simulink model "sampleModel160"  (R2021b)
settings: Solver=VariableStepAuto  StartTime=0.0  StopTime=10.0  RelTol=1e-3
undefined symbols (not defined in the file or in its folder): DiscIntNeverNeededParam, Newton, Raphson
libraries: simulink x16, slpidlib x1
settings Model: Creator=user  LastModifiedBy=user

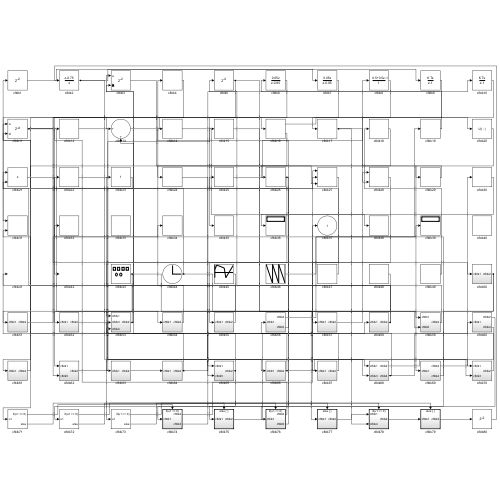
[thumbnail: Simulink's stored preview of the top-level diagram]
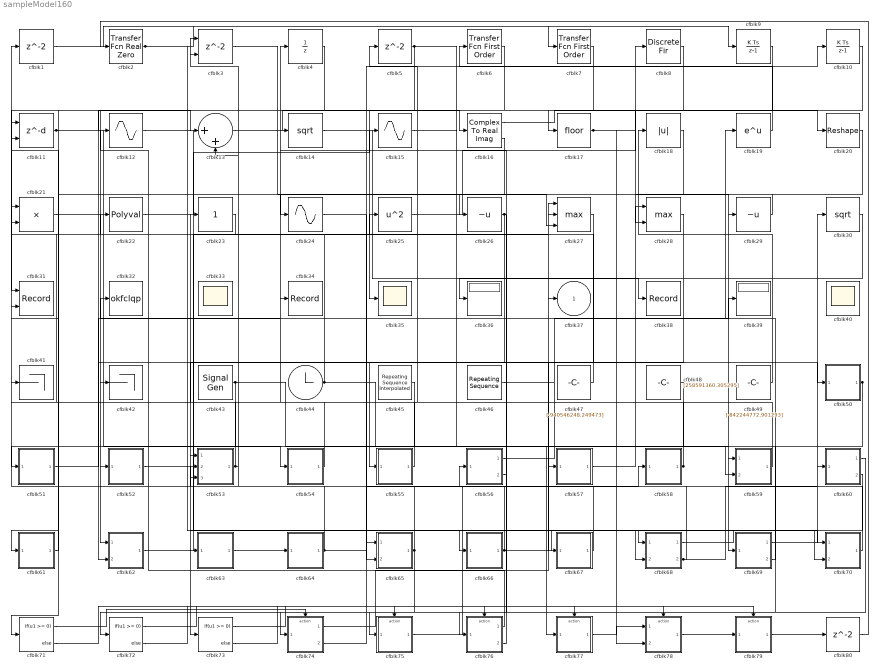
== system sampleModel160 ==
  cfblk1 : Delay  SampleTime=1
  cfblk10 : DiscreteIntegrator  ICPrevOutput=DiscIntNeverNeededParam  ICPrevScaledInput=DiscIntNeverNeededParam
  cfblk11 : Delay  DelayLengthSource=Input port  SampleTime=1
      settings: InputPortMap=u0,p1
  cfblk12 : Sin  TimeSource=Use external signal  SampleTime=0
  cfblk13 : Sum  Inputs=|++
  cfblk14 : Sqrt  SaturateOnIntegerOverflow=on
  cfblk15 : Sin  TimeSource=Use external signal  SampleTime=0
  cfblk16 : ComplexToRealImag
  cfblk17 : Rounding
  cfblk18 : Abs
  cfblk19 : Math  SaturateOnIntegerOverflow=on
  cfblk2 : simulink/Discrete/Transfer Fcn Real Zero  ZeroZ=0.75  ICPrevInput=0.0  DoSatur=off
      settings: SourceProductBaseCode=SL
  cfblk20 : Reshape
  cfblk21 : Product  Inputs=**
  cfblk22 : Polyval  Coefs=[ +2.081618890e-019, -1.441693666e-014, +4.719686976e-010, -8.536869453e-006, +1.621573104e-001, -8.087801117e+001 ]
  cfblk23 : simulink/Math Operations/Slider Gain  gain=1  low=0  high=2
  cfblk24 : Sin  TimeSource=Use external signal  SampleTime=0
  cfblk25 : Math  Operator=square  SaturateOnIntegerOverflow=on
  cfblk26 : UnaryMinus
  cfblk27 : MinMax  Function=max  Inputs=3
  cfblk28 : MinMax  Function=max  Inputs=2
  cfblk29 : UnaryMinus
  cfblk3 : Delay  ShowEnablePort=on  SampleTime=1
      settings: InputPortMap=u0,e6
  cfblk30 : Sqrt  SaturateOnIntegerOverflow=on
  cfblk31 : Record  FileSettingsInternal="{\"entries\":[{\"content\":{\"excelSettings\":{\"content\":{},\"type\":\"Streamout.ExcelSettings\"}},\"type\":\"Streamout.FileSettingStorage\",\"uuid\":\"c413c589-d2ce-436c-aaba-4ffc6c089058\"}],\"packageUris\":[\"http://schema.mathworks.com/mf0/streamout_blocks/R2020a\"],\"version\":\"1.0\"}"  Layout=[1 1]  SignalsInternal="{\"entries\":[{\"content\":{\"signals\":[{\"content\":{\"blockPath\":[\"sampleModel160/cfblk31\"],\"channel\":[],\"dimensions\":[1],\"domain\":\"sampleModel160/cfblk31\",\"lineColor\":\"#a2142f\",\"plots\":[1],\"port\":1,\"sid\":[\"\"],\"signalID\":6037,\"signalName\":\"cfblk10\"},\"type\":\"RecordBlkView.Signal\",\"uuid\":\"72857fe4-462d-486d-a3e4-3c395ee845b6\"},{\"content\":{\"blockPath\":[\"sampleModel160/cfblk31\"],\"channel\":[],\"dimensions\":[1],\"domain\":\"sampleModel160/cfblk31\",\"lineColor\":\"#139fff\",\"plots\":[1],\"port\":2,\"sid\":[\"\"],\"signalID\":6041,\"signalName\":\"cfblk61\"},\"type\":\"RecordBlkView.Signal\",\"uuid\":\"d5c775f5-053a-4779-9e26-d54423a1e3c8\"}]},\"type\":\"RecordBlkView.InputSignals\",\"uuid\":\"1cc1dd8b-340d-4e21-9a8e-fa59a4d45196\"}],\"packageUris\":[\"http://schema.mathworks.com/mf0/streamout_blocks/R2020a\"],\"version\":\"1.0\"}"  VisualizationBindings="{\"xyplotplugin\":{\"info\":[{\"series\":[{\"bindingParametersList\":[{\"parameter\":\"X-Axis\",\"signalID\":6037,\"signalName\":\"cfblk10\"},{\"parameter\":\"Y-Axis\",\"signalID\":6041,\"signalName\":\"cfblk61\"}],\"seriesID\":10105}],\"subplotID\":1}]}}"  CompatibilityTag=XY
  cfblk32 : ToWorkspace  VariableName=okfclqp  SaveFormat=Timeseries  SampleTime=-1
  cfblk33 : Scope
      settings: Floating=on
  cfblk34 : Record  FileSettingsInternal="{\"entries\":[{\"content\":{\"excelSettings\":{\"content\":{},\"type\":\"Streamout.ExcelSettings\"}},\"type\":\"Streamout.FileSettingStorage\",\"uuid\":\"c9e76eac-59f3-42f9-ba3c-d666261c6b06\"}],\"packageUris\":[\"http://schema.mathworks.com/mf0/streamout_blocks/R2020a\"],\"version\":\"1.0\"}"  SignalsInternal="{\"entries\":[{\"content\":{\"signals\":[{\"content\":{\"blockPath\":[\"sampleModel160/cfblk34\"],\"channel\":[],\"dimensions\":[1],\"domain\":\"sampleModel160/cfblk34\",\"lineColor\":\"#fe330a\",\"plots\":[1],\"port\":1,\"sid\":[\"\"],\"signalID\":6045,\"signalName\":\"cfblk51\"},\"type\":\"RecordBlkView.Signal\",\"uuid\":\"385a5dff-ef78-469a-be59-ea6837f228a9\"}]},\"type\":\"RecordBlkView.InputSignals\",\"uuid\":\"b764ceec-8da9-4fc6-845a-cebcb7dbad93\"}],\"packageUris\":[\"http://schema.mathworks.com/mf0/streamout_blocks/R2020a\"],\"version\":\"1.0\"}"  VisualizationBindings="{\"sparklinesplugin\":{\"info\":[{\"bindingParametersList\":[],\"subplotID\":1}]}}"
  cfblk35 : Scope
  cfblk36 : Display
  cfblk38 : Record  FileSettingsInternal="{\"entries\":[{\"content\":{\"excelSettings\":{\"content\":{},\"type\":\"Streamout.ExcelSettings\"}},\"type\":\"Streamout.FileSettingStorage\",\"uuid\":\"a9748414-4318-452a-bfbb-77e6d7b29a13\"}],\"packageUris\":[\"http://schema.mathworks.com/mf0/streamout_blocks/R2020a\"],\"version\":\"1.0\"}"  SignalsInternal="{\"entries\":[{\"content\":{\"signals\":[{\"content\":{\"blockPath\":[\"sampleModel160/cfblk38\"],\"channel\":[],\"dimensions\":[1],\"domain\":\"sampleModel160/cfblk38\",\"lineColor\":\"#22b573\",\"plots\":[1],\"port\":1,\"sid\":[\"\"],\"signalID\":6049,\"signalName\":\"cfblk14\"},\"type\":\"RecordBlkView.Signal\",\"uuid\":\"85378120-5b17-4b37-8955-e146c021a7fe\"}]},\"type\":\"RecordBlkView.InputSignals\",\"uuid\":\"a0d2f558-881a-48b2-8250-b54130961238\"}],\"packageUris\":[\"http://schema.mathworks.com/mf0/streamout_blocks/R2020a\"],\"version\":\"1.0\"}"  VisualizationBindings="{\"sparklinesplugin\":{\"info\":[{\"bindingParametersList\":[],\"subplotID\":1}]}}"
  cfblk39 : Display
  cfblk4 : UnitDelay  HasFrameUpgradeWarning=on
  cfblk40 : Scope
      settings: Floating=on
  cfblk41 : Terminator
  cfblk42 : Terminator
  cfblk43 : SignalGenerator  Amplitude=[899162175.269200]
  cfblk44 : Clock
  cfblk45 : simulink/Sources/Repeating Sequence Interpolated  OutValues=[358173877.356189, 804234155.488900, 502386956.729002, -523743488.961026, 763410355.711706]  TimeValues=[0 0.1 0.5 0.6 1].'  LookUpMeth=Interpolation-Use End Values  tsamp=0.01  OutMin=[]  OutMax=[]  OutDataTypeStr=double  OutputDataTypeScalingMode=double  OutDataType=fixdt(0,8)  OutScaling=2^-10
  cfblk46 : simulink/Sources/Repeating Sequence  rep_seq_t=[0 2]  rep_seq_y=[661275798.341106, -980251664.687721]
  cfblk47 : Constant  Value=[-940546248.249473]  SampleTime=1
  cfblk48 : Constant  Value=[258591360.305295]  SampleTime=1
  cfblk49 : Constant  Value=[-842244772.901293]  SampleTime=1
  cfblk5 : Delay  SampleTime=1
  cfblk50 : Subsystem
  cfblk51 : Subsystem
  cfblk52 : Subsystem
  cfblk53 : Subsystem
  cfblk54 : Subsystem
  cfblk55 : Subsystem
  cfblk56 : Subsystem
  cfblk57 : Subsystem
  cfblk58 : Subsystem
  cfblk59 : Subsystem
  cfblk6 : simulink/Discrete/Transfer Fcn First Order  PoleZ=0.95  ICPrevOutput=0.0  DoSatur=off
  cfblk60 : Subsystem
  cfblk61 : Subsystem
  cfblk62 : Subsystem
  cfblk63 : Subsystem
  cfblk64 : Subsystem
  cfblk65 : Subsystem
  cfblk66 : Subsystem
  cfblk67 : Subsystem
  cfblk68 : Subsystem
  cfblk69 : Subsystem
  cfblk7 : simulink/Discrete/Transfer Fcn First Order  PoleZ=0.95  ICPrevOutput=0.0  DoSatur=off
  cfblk70 : Subsystem
  cfblk71 : If  IfExpression=u1 >= 0  SampleTime=1
  cfblk72 : If  IfExpression=u1 >= 0  SampleTime=1
  cfblk73 : If  IfExpression=u1 >= 0  SampleTime=1
  cfblk74 : Subsystem  TreatAsAtomicUnit=on
  cfblk75 : Subsystem  TreatAsAtomicUnit=on
  cfblk76 : Subsystem  TreatAsAtomicUnit=on
  cfblk77 : Subsystem  TreatAsAtomicUnit=on
  cfblk78 : Subsystem  TreatAsAtomicUnit=on
  cfblk79 : Subsystem  TreatAsAtomicUnit=on
  cfblk8 : DiscreteFir  SampleTime=1
  cfblk80 : Delay  SampleTime=1
  cfblk9 : DiscreteIntegrator  ICPrevOutput=DiscIntNeverNeededParam  ICPrevScaledInput=DiscIntNeverNeededParam
  cfblk37 : Outport
  wires:
  cfblk20/1 -> cfblk69/1(cfblk1)
  cfblk50/1(cfblk2) -> cfblk75/1(cfblk1), cfblk51/1(cfblk1)
  cfblk14/1 -> cfblk38/1
  cfblk49/1 -> cfblk18/1
  cfblk6/1 -> cfblk35/1
  cfblk57/1(cfblk2) -> cfblk28/1
  cfblk13/1 -> cfblk16/1
  cfblk67/1(cfblk2) -> cfblk56/1(cfblk1)
  cfblk1/1 -> cfblk7/1
  cfblk19/1 -> cfblk6/1
  cfblk74/1(cfblk2) -> cfblk27/1
  cfblk62/1(cfblk2) -> cfblk27/2
  cfblk69/1(cfblk2) -> cfblk30/1
  cfblk21/1 -> cfblk62/1(cfblk1)
  cfblk60/1(cfblk2) -> cfblk74/1(cfblk1)
  cfblk24/1 -> cfblk65/1(cfblk1)
  cfblk25/1 -> cfblk8/1
  cfblk70/1(cfblk2) -> cfblk1/1
  cfblk9/1 -> cfblk28/2
  cfblk10/1 -> cfblk31/1
  cfblk2/1 -> cfblk9/1, cfblk68/2(cfblk3)
  cfblk11/1 -> cfblk54/1(cfblk1), cfblk13/1, cfblk50/1(cfblk1)
  cfblk54/1(cfblk2) -> cfblk4/1
  cfblk75/1(cfblk2) -> cfblk37/1
  cfblk3/1 -> cfblk27/3
  cfblk29/1 -> cfblk24/1
  cfblk12/1 -> cfblk66/1(cfblk1)
  cfblk17/1 -> cfblk29/1, cfblk78/2(cfblk4)
  cfblk66/1(cfblk2) -> cfblk68/1(cfblk1), cfblk3/1
  cfblk60/2(cfblk4) -> cfblk73/1
  cfblk43/1 -> cfblk52/1(cfblk1), cfblk77/1(cfblk1)
  cfblk28/1 -> cfblk55/1(cfblk1)
  cfblk30/1 -> cfblk36/1
  cfblk77/1(cfblk2) -> cfblk78/1(cfblk1)
  cfblk18/1 -> cfblk26/1
  cfblk74/2(cfblk3) -> cfblk58/1(cfblk1)
  cfblk7/1 -> cfblk71/1
  cfblk8/1 -> cfblk17/1
  cfblk4/1 -> cfblk42/1
  cfblk51/1(cfblk2) -> cfblk34/1
  cfblk78/1(cfblk2) -> cfblk79/1(cfblk1)
  cfblk56/1(cfblk2) -> cfblk19/1
  cfblk27/1 -> cfblk67/1(cfblk1)
  cfblk46/1 -> cfblk39/1
  cfblk68/1(cfblk2) -> cfblk70/1(cfblk1)
  cfblk68/2(cfblk4) -> cfblk60/1(cfblk1), cfblk53/3(cfblk4)
  cfblk53/1(cfblk2) -> cfblk21/1, cfblk3/2
  cfblk64/1(cfblk2) -> cfblk10/1, cfblk53/2(cfblk3)
  cfblk63/1(cfblk2) -> cfblk64/1(cfblk1)
  cfblk59/1(cfblk2) -> cfblk41/1
  cfblk23/1 -> cfblk21/2
  cfblk22/1 -> cfblk15/1
  cfblk69/2(cfblk4) -> cfblk32/1
  cfblk61/1(cfblk2) -> cfblk31/2
  cfblk52/1(cfblk2) -> cfblk70/2(cfblk3)
  cfblk44/1 -> cfblk57/1(cfblk1), cfblk11/2
  cfblk26/1 -> cfblk76/1(cfblk1), cfblk53/1(cfblk1)
  cfblk55/1(cfblk2) -> cfblk23/1
  cfblk45/1 -> cfblk65/2(cfblk5)
  cfblk76/1(cfblk2) -> cfblk12/1
  cfblk48/1 -> cfblk63/1(cfblk1)
  cfblk56/2(cfblk3) -> cfblk22/1
  cfblk65/1(cfblk2) -> cfblk11/1, cfblk72/1
  cfblk16/1 -> cfblk20/1
  cfblk16/2 -> cfblk61/1(cfblk1)
  cfblk58/1(cfblk2) -> cfblk5/1, cfblk13/2
  cfblk76/2(cfblk5) -> cfblk14/1
  cfblk47/1 -> cfblk25/1
  cfblk15/1 -> cfblk59/1(cfblk1)
  cfblk5/1 -> cfblk62/2(cfblk5), cfblk59/2(cfblk5)
  cfblk71/1 -> cfblk74/Action
  cfblk71/2 -> cfblk75/Action
  cfblk72/1 -> cfblk76/Action
  cfblk72/2 -> cfblk77/Action
  cfblk73/1 -> cfblk78/Action
  cfblk73/2 -> cfblk79/Action
  cfblk79/1(cfblk2) -> cfblk80/1
  cfblk80/1 -> cfblk2/1

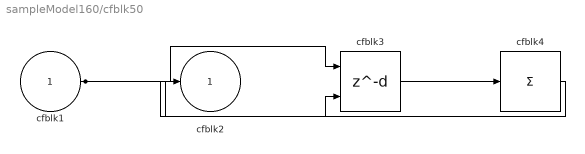
== system sampleModel160/cfblk50 ==
  cfblk1 : Inport
  cfblk3 : Delay  DelayLengthSource=Input port  SampleTime=1
      settings: InputPortMap=u0,p1
  cfblk4 : Sum  Inputs=+
  cfblk2 : Outport
  wires:
  cfblk1/1 -> cfblk3/1, cfblk3/2
  cfblk4/1 -> cfblk2/1
  cfblk3/1 -> cfblk4/1

== system sampleModel160/cfblk51 ==
  cfblk1 : Inport
  cfblk3 : Reshape
  cfblk2 : Outport
  wires:
  cfblk1/1 -> cfblk3/1
  cfblk3/1 -> cfblk2/1

== system sampleModel160/cfblk52 ==
  cfblk1 : Inport
  cfblk3 : simulink/Discrete/Tapped Delay  vinit=0.0  samptime=-1  NumDelays=1  DelayOrder=Oldest  includeCurrent=off
  cfblk2 : Outport
  wires:
  cfblk1/1 -> cfblk3/1
  cfblk3/1 -> cfblk2/1

== system sampleModel160/cfblk53 ==
  cfblk1 : Inport
  cfblk3 : Inport  Port=2
  cfblk4 : Inport  Port=3
  cfblk2 : Outport
  wires:
  cfblk1/1 -> cfblk2/1

== system sampleModel160/cfblk54 ==
  cfblk1 : Inport
  cfblk3 : Math  Operator=rem  SaturateOnIntegerOverflow=on
  cfblk2 : Outport
  wires:
  cfblk1/1 -> cfblk3/1, cfblk3/2
  cfblk3/1 -> cfblk2/1

== system sampleModel160/cfblk55 ==
  cfblk1 : Inport
  cfblk3 : ComplexToMagnitudeAngle
  cfblk2 : Outport
  wires:
  cfblk1/1 -> cfblk3/1
  cfblk3/1 -> cfblk2/1

== system sampleModel160/cfblk56 ==
  cfblk1 : Inport
  cfblk2 : Outport
  cfblk3 : Outport  Port=2
  wires:
  cfblk1/1 -> cfblk2/1, cfblk3/1

== system sampleModel160/cfblk57 ==
  cfblk1 : Inport
  cfblk3 : simulink/Discrete/Tapped Delay  vinit=0.0  samptime=-1  NumDelays=1  DelayOrder=Oldest  includeCurrent=off
  cfblk2 : Outport
  wires:
  cfblk1/1 -> cfblk3/1
  cfblk3/1 -> cfblk2/1

== system sampleModel160/cfblk58 ==
  cfblk1 : Inport
  cfblk3 : simulink/Discrete/Transfer Fcn Real Zero  ZeroZ=0.75  ICPrevInput=0.0  DoSatur=off
      settings: SourceProductBaseCode=SL
  cfblk2 : Outport
  wires:
  cfblk1/1 -> cfblk3/1
  cfblk3/1 -> cfblk2/1

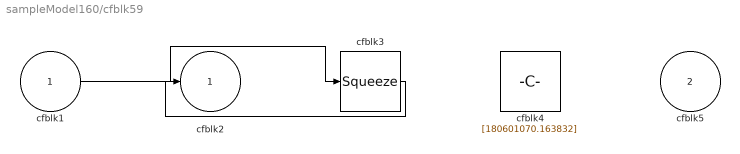
== system sampleModel160/cfblk59 ==
  cfblk1 : Inport
  cfblk5 : Inport  Port=2
  cfblk3 : Squeeze
  cfblk4 : Constant  Value=[180601070.163832]  SampleTime=1
  cfblk2 : Outport
  wires:
  cfblk1/1 -> cfblk3/1
  cfblk3/1 -> cfblk2/1

== system sampleModel160/cfblk60 ==
  cfblk1 : Inport
  cfblk3 : slpidlib/PID Controller (2DOF)  Controller=PID  Form=Parallel  TimeDomain=Discrete-time  UseExternalTs=off  SampleTime=1  IntegratorMethod=Forward Euler  FilterMethod=Forward Euler  ControllerParametersSource=internal  P=1  I=1  D=0  UseFilter=on  N=100  b=1  c=1  TunerSelectOption=Transfer Function Based (PID Tuner App)  InitialConditionSource=internal  InitialConditionForIntegrator=0  InitialConditionForFilter=0  DifferentiatorICPrevScaledInput=0  ExternalReset=none  TrackingMode=off  Kt=1  LimitOutput=off  SatLimitsSource=internal  UpperSaturationLimit=inf  LowerSaturationLimit=-inf  LinearizeAsGain=off  AntiWindupMode=none  Kb=1  POutMin=[]  POutMax=[]  IOutMin=[]  IOutMax=[]  DOutMin=[]  DOutMax=[]  NOutMin=[]  NOutMax=[]  bOutMin=[]  bOutMax=[]  cOutMin=[]  cOutMax=[]  SumOutMin=[]  SumOutMax=[]  SaturationOutMin=[]  SaturationOutMax=[]  PParamMin=[]  PParamMax=[]  IParamMin=[]  IParamMax=[]  DParamMin=[]  DParamMax=[]  NParamMin=[]  NParamMax=[]  bParamMin=[]  bParamMax=[]  cParamMin=[]  cParamMax=[]  KbParamMin=[]  KbParamMax=[]  KtParamMin=[]  KtParamMax=[]  KbOutMin=[]  KbOutMax=[]  KtOutMin=[]  KtOutMax=[]  IntegratorOutMin=[]  IntegratorOutMax=[]  FilterOutMin=[]  FilterOutMax=[]  SumI1OutMin=[]  SumI1OutMax=[]  SumI2OutMin=[]  SumI2OutMax=[]  SumI3OutMin=[]  SumI3OutMax=[]  SumI4OutMin=[]  SumI4OutMax=[]  SumDOutMin=[]  SumDOutMax=[]  Sum1OutMin=[]  Sum1OutMax=[]  Sum2OutMin=[]  Sum2OutMax=[]  Sum3OutMin=[]  Sum3OutMax=[]  DifferentiatorOutMin=[]  DifferentiatorOutMax=[]  FilterDiffOutCoefMin=[]  FilterDiffOutCoefMax=[]  ReciprocalOutMin=[]  ReciprocalOutMax=[]  SumDenOutMin=[]  SumDenOutMax=[]  SumNumOutMin=[]  SumNumOutMax=[]  DivideOutMin=[]  DivideOutMax=[]  UdiffTsProdOutMin=[]  UdiffTsProdOutMax=[]  NTsProdOutMin=[]  NTsProdOutMax=[]  UintegralTsProdOutMin=[]  UintegralTsProdOutMax=[]  UngainTsProdOutMin=[]  UngainTsProdOutMax=[]  IntegratorContinuousStateAttributes=''  IntegratorStateMustResolveToSignalObject=off  IntegratorRTWStateStorageClass=Auto  FilterContinuousStateAttributes=''  FilterStateMustResolveToSignalObject=off  FilterRTWStateStorageClass=Auto  ParallelPVariant=InternalParameters  IdealPVariant=Disabled  IVariant=InternalParameters  DVariant=InternalParameters  bVariant=InternalParameters  cVariant=InternalParameters  IntegratorVariant=Discrete  SatVariant=Disabled  AWVariant=Passthrough  PCopyVariant=Disabled  TRVariant=Disabled  FdbkBlocksVariant=Forward  IdealPFdbkVariant=Disabled  SatFdbkVariant=Disabled  DerivativeFilterVariant=ForwardEulerFilter  NVariant=InternalParameters  NCopyVariant=Disabled  FilterICVariant=InternalICsFilter  IntegratorICVariant=InternalICs  ExternalResetVariant=Disabled  TRSumVariant=Passthrough  SumFdbkVariant=Disabled  SumVariant=Sum_PID  TsampFilterVariant=InternalTs  TsampNgainVariant=Passthrough  TsampIntegralVariant=Passthrough  ExternalSaturationOutDataTypeStr=Inherit: Same as second input
      settings: SourceProductBaseCode=SL
  cfblk2 : Outport
  cfblk4 : Outport  Port=2
  wires:
  cfblk3/1 -> cfblk4/1
  cfblk1/1 -> cfblk2/1, cfblk3/1, cfblk3/2

== system sampleModel160/cfblk61 ==
  cfblk1 : Inport
  cfblk3 : simulink/Discrete/Transfer Fcn Lead or Lag  PoleZ=0.95  ZeroZ=0.75  ICPrevOutput=0.0  ICPrevInput=0.0  DoSatur=off
      settings: SourceProductBaseCode=SL
  cfblk4 : Constant  Value=[-66173144.948453]  SampleTime=1
  cfblk2 : Outport
  wires:
  cfblk4/1 -> cfblk2/1
  cfblk1/1 -> cfblk3/1

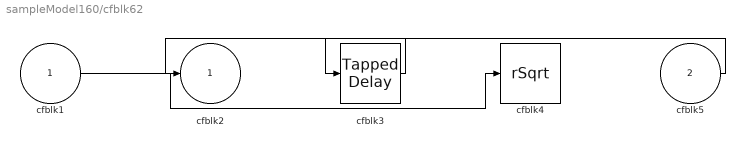
== system sampleModel160/cfblk62 ==
  cfblk1 : Inport
  cfblk5 : Inport  Port=2
  cfblk3 : simulink/Discrete/Tapped Delay  vinit=0.0  samptime=-1  NumDelays=1  DelayOrder=Oldest  includeCurrent=off
  cfblk4 : Sqrt  Operator=rSqrt  AlgorithmType=Newton-Raphson  SaturateOnIntegerOverflow=on
  cfblk2 : Outport
  wires:
  cfblk5/1 -> cfblk3/1
  cfblk1/1 -> cfblk4/1
  cfblk3/1 -> cfblk2/1

== system sampleModel160/cfblk63 ==
  cfblk1 : Inport
  cfblk3 : Sum  Inputs=+-
  cfblk2 : Outport
  wires:
  cfblk1/1 -> cfblk3/1, cfblk3/2
  cfblk3/1 -> cfblk2/1

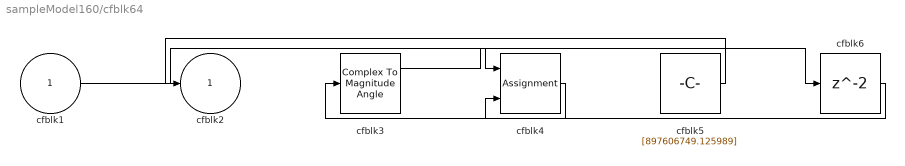
== system sampleModel160/cfblk64 ==
  cfblk1 : Inport
  cfblk3 : ComplexToMagnitudeAngle
  cfblk4 : Assignment  DiagnosticForDimensions=Warning  IndexOptions=Index vector (dialog)  Indices=1  OutputSizes=1
  cfblk5 : Constant  Value=[897606749.125989]  SampleTime=1
  cfblk6 : Delay  SampleTime=1
  cfblk2 : Outport
  wires:
  cfblk1/1 -> cfblk4/1
  cfblk4/1 -> cfblk3/1
  cfblk5/1 -> cfblk2/1
  cfblk3/1 -> cfblk6/1
  cfblk6/1 -> cfblk4/2

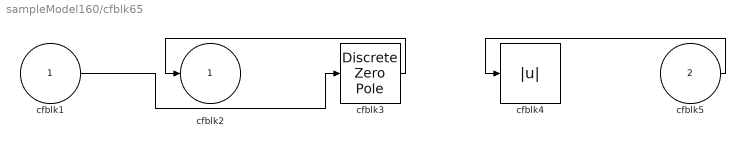
== system sampleModel160/cfblk65 ==
  cfblk1 : Inport
  cfblk5 : Inport  Port=2
  cfblk3 : DiscreteZeroPole  Poles=[0 0.5]  Gain=1
  cfblk4 : Abs
  cfblk2 : Outport
  wires:
  cfblk5/1 -> cfblk4/1
  cfblk3/1 -> cfblk2/1
  cfblk1/1 -> cfblk3/1

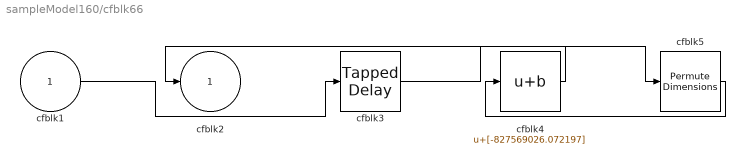
== system sampleModel160/cfblk66 ==
  cfblk1 : Inport
  cfblk3 : simulink/Discrete/Tapped Delay  vinit=0.0  samptime=-1  NumDelays=1  DelayOrder=Oldest  includeCurrent=off
  cfblk4 : Bias  Bias=[-827569026.072197]
  cfblk5 : PermuteDimensions
  cfblk2 : Outport
  wires:
  cfblk4/1 -> cfblk2/1
  cfblk5/1 -> cfblk4/1
  cfblk1/1 -> cfblk3/1
  cfblk3/1 -> cfblk5/1

== system sampleModel160/cfblk67 ==
  cfblk1 : Inport
  cfblk3 : simulink/Discrete/Difference  ICPrevInput=0.0  OutMin=[]  OutMax=[]  OutDataTypeStr=Inherit: Inherit via back propagation  OutDataType=fixdt(1, 16)  OutScaling=2^-10  DoSatur=off
  cfblk2 : Outport
  wires:
  cfblk1/1 -> cfblk2/1, cfblk3/1

== system sampleModel160/cfblk68 ==
  cfblk1 : Inport
  cfblk3 : Inport  Port=2
  cfblk2 : Outport
  cfblk4 : Outport  Port=2
  wires:
  cfblk3/1 -> cfblk2/1
  cfblk1/1 -> cfblk4/1

== system sampleModel160/cfblk69 ==
  cfblk1 : Inport
  cfblk3 : DiscreteStateSpace
  cfblk2 : Outport
  cfblk4 : Outport  Port=2
  wires:
  cfblk3/1 -> cfblk2/1
  cfblk1/1 -> cfblk4/1, cfblk3/1

== system sampleModel160/cfblk70 ==
  cfblk1 : Inport
  cfblk3 : Inport  Port=2
  cfblk2 : Outport
  wires:
  cfblk3/1 -> cfblk2/1

== system sampleModel160/cfblk74 ==
  cfblk1 : Inport
  Action Port : ActionPort  ActionPortLabel=if(u1 >= 0)
  cfblk2 : Outport
  cfblk3 : Outport  Port=2
  wires:
  cfblk1/1 -> cfblk2/1, cfblk3/1

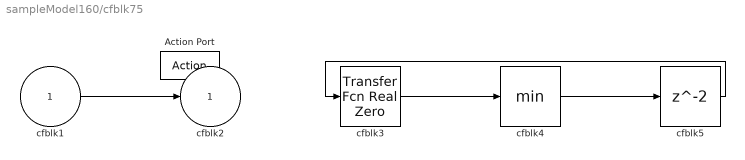
== system sampleModel160/cfblk75 ==
  cfblk1 : Inport
  Action Port : ActionPort  ActionPortLabel=else
  cfblk3 : simulink/Discrete/Transfer Fcn Real Zero  ZeroZ=0.75  ICPrevInput=0.0  DoSatur=off
      settings: SourceProductBaseCode=SL
  cfblk4 : MinMax
  cfblk5 : Delay
  cfblk2 : Outport
  wires:
  cfblk3/1 -> cfblk4/1
  cfblk1/1 -> cfblk2/1
  cfblk4/1 -> cfblk5/1
  cfblk5/1 -> cfblk3/1

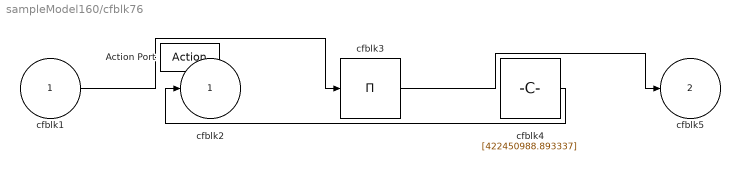
== system sampleModel160/cfblk76 ==
  cfblk1 : Inport
  Action Port : ActionPort  ActionPortLabel=if(u1 >= 0)
  cfblk3 : Product  Inputs=*
  cfblk4 : Constant  Value=[422450988.893337]  SampleTime=1
  cfblk2 : Outport
  cfblk5 : Outport  Port=2
  wires:
  cfblk4/1 -> cfblk2/1
  cfblk3/1 -> cfblk5/1
  cfblk1/1 -> cfblk3/1

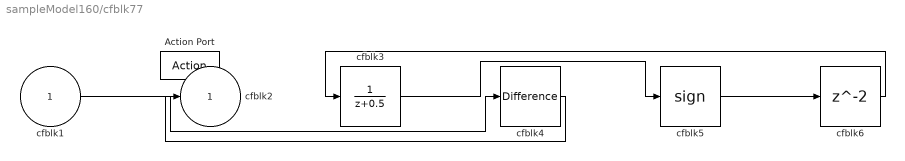
== system sampleModel160/cfblk77 ==
  cfblk1 : Inport
  Action Port : ActionPort  ActionPortLabel=else
  cfblk3 : DiscreteTransferFcn
  cfblk4 : simulink/Discrete/Difference  ICPrevInput=0.0  OutMin=[]  OutMax=[]  OutDataTypeStr=Inherit: Inherit via back propagation  OutDataType=fixdt(1, 16)  OutScaling=2^-10  DoSatur=off
  cfblk5 : Signum
  cfblk6 : Delay
  cfblk2 : Outport
  wires:
  cfblk1/1 -> cfblk4/1
  cfblk4/1 -> cfblk2/1
  cfblk3/1 -> cfblk5/1
  cfblk5/1 -> cfblk6/1
  cfblk6/1 -> cfblk3/1

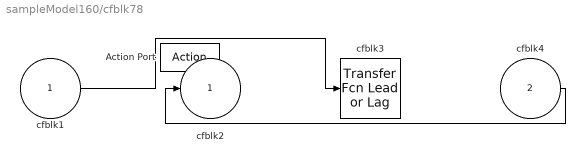
== system sampleModel160/cfblk78 ==
  cfblk1 : Inport
  cfblk4 : Inport  Port=2
  Action Port : ActionPort  ActionPortLabel=if(u1 >= 0)
  cfblk3 : simulink/Discrete/Transfer Fcn Lead or Lag  PoleZ=0.95  ZeroZ=0.75  ICPrevOutput=0.0  ICPrevInput=0.0  DoSatur=off
      settings: SourceProductBaseCode=SL
  cfblk2 : Outport
  wires:
  cfblk4/1 -> cfblk2/1
  cfblk1/1 -> cfblk3/1

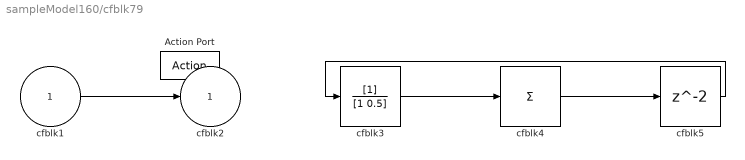
== system sampleModel160/cfblk79 ==
  cfblk1 : Inport
  Action Port : ActionPort  ActionPortLabel=else
  cfblk3 : DiscreteFilter
  cfblk4 : Sum  Inputs=+
  cfblk5 : Delay
  cfblk2 : Outport
  wires:
  cfblk1/1 -> cfblk2/1
  cfblk3/1 -> cfblk4/1
  cfblk4/1 -> cfblk5/1
  cfblk5/1 -> cfblk3/1
